simulink model "matlab_function"  (R2017b)
settings: Solver=VariableStepAuto  StartTime=1960  StopTime=2010  RelTol=1e-3
settings Model: Creator=jim  LastModifiedBy=jim

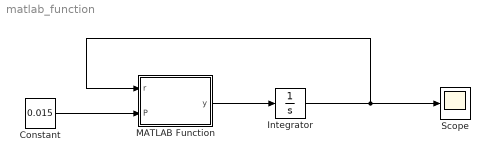
== system matlab_function ==
  Constant : Constant  Value=0.015
  Integrator : Integrator  InitialCondition=3000
  MATLAB Function : MATLAB Function  TreatAsAtomicUnit=on
  Scope : Scope
  wires:
  MATLAB Function/1(y) -> Integrator/1
  Integrator/1 -> Scope/1, MATLAB Function/1(r)
  Constant/1 -> MATLAB Function/2(P)

== matlab function matlab_function/MATLAB Function ==
  data: r input; P input; y output
function y = fcn(r, P)

y = r * P;
